simulink model "P702_NI_SoftECU"  (R2019a)
settings: Solver=ode1  StartTime=0.0  StopTime=Inf  FixedStep=0.001  RelTol=1e-3  EnableMultiTasking=on
PreLoadFcn:
  | run '.\VeriStand_BlockSet\NIVeriStandAddPaths.m'
undefined symbols (not defined in the file or in its folder): magnitude
libraries: simulink x83, simulink_extras x1
(part 73 of 76)

== system P702_NI_SoftECU/Output/Subsystem1/CAN_Signal/GWM/RCM/RCMStatusMessage2_FD1_4C ==
  in_port : Inport
  EDRTriggerEvntSync : Terminator
  FirstRowBuckleDriver : Terminator
  FirstRowBuckleMid : Terminator
  FirstRowBucklePsngr : Terminator
  PassRstrnInd_Req : Terminator
  PsngrFmidDetct_D_Actl : Terminator
  PsngrFrntDetct_D_Actl : Terminator
  RILReq : Terminator
  RstrnImpactEvntStatus : Terminator
  RstrnPsngrOn_D_Stat : Terminator
  SecondRowBuckleDriver : Terminator
  SecondRowBuckleMid : Terminator
  SecondRowBucklePsngr : Terminator
  ThirdRowBuckleDriver : Terminator
  ThirdRowBuckleMid : Terminator
  ThirdRowBucklePsngr : Terminator
  bus_selector : BusSelector  OutputSignals=EDRTriggerEvntSync,FirstRowBuckleDriver,FirstRowBuckleMid,FirstRowBucklePsngr,PassRstrnInd_Req,PsngrFmidDetct_D_Actl,PsngrFrntDetct_D_Actl,RILReq,RstrnImpactEvntStatus,RstrnPsngrOn_D_Stat,SecondRowBuckleDriver,SecondRowBuckleMid,SecondRowBucklePsngr,ThirdRowBuckleDriver,ThirdRowBuckleMid,ThirdRowBucklePsngr
  wires:
  in_port/1 -> bus_selector/1  "Subsystem1"
  bus_selector/1 -> EDRTriggerEvntSync/1  "<EDRTriggerEvntSync>"
  bus_selector/2 -> FirstRowBuckleDriver/1  "<FirstRowBuckleDriver>"
  bus_selector/3 -> FirstRowBuckleMid/1  "<FirstRowBuckleMid>"
  bus_selector/4 -> FirstRowBucklePsngr/1  "<FirstRowBucklePsngr>"
  bus_selector/5 -> PassRstrnInd_Req/1  "<PassRstrnInd_Req>"
  bus_selector/6 -> PsngrFmidDetct_D_Actl/1  "<PsngrFmidDetct_D_Actl>"
  bus_selector/7 -> PsngrFrntDetct_D_Actl/1  "<PsngrFrntDetct_D_Actl>"
  bus_selector/8 -> RILReq/1  "<RILReq>"
  bus_selector/9 -> RstrnImpactEvntStatus/1  "<RstrnImpactEvntStatus>"
  bus_selector/10 -> RstrnPsngrOn_D_Stat/1  "<RstrnPsngrOn_D_Stat>"
  bus_selector/11 -> SecondRowBuckleDriver/1  "<SecondRowBuckleDriver>"
  bus_selector/12 -> SecondRowBuckleMid/1  "<SecondRowBuckleMid>"
  bus_selector/13 -> SecondRowBucklePsngr/1  "<SecondRowBucklePsngr>"
  bus_selector/14 -> ThirdRowBuckleDriver/1  "<ThirdRowBuckleDriver>"
  bus_selector/15 -> ThirdRowBuckleMid/1  "<ThirdRowBuckleMid>"
  bus_selector/16 -> ThirdRowBucklePsngr/1  "<ThirdRowBucklePsngr>"

== system P702_NI_SoftECU/Output/Subsystem1/CAN_Signal/GWM/SCCM/Steering_Data_FD1_83 ==
  in_port : Inport
  AccButtnGapDecPress : Terminator
  AccButtnGapIncPress : Terminator
  AccButtnGapTogglePress : Terminator
  AhbStat_B_Dsply : Terminator
  AslButtnOnOffCnclPress : Terminator
  AslButtnOnOffPress : Terminator
  CcAslButtnCnclPress : Terminator
  CcAslButtnCnclResPress : Terminator
  CcAslButtnDeny_B_Actl : Terminator
  CcAslButtnIndxDecPress : Terminator
  CcAslButtnIndxIncPress : Terminator
  CcAslButtnOffCnclPress : Terminator
  CcAslButtnOnOffCncl : Terminator
  CcAslButtnOnPress : Terminator
  CcAslButtnResDecPress : Terminator
  CcAslButtnResIncPress : Terminator
  CcAslButtnSetDecPress : Terminator
  CcAslButtnSetIncPress : Terminator
  CcAslButtnSetPress : Terminator
  CcAsllButtnResPress : Terminator
  CcButtnOffPress : Terminator
  CcButtnOnOffCnclPress : Terminator
  CcButtnOnOffPress : Terminator
  CcButtnOnPress : Terminator
  HeadLghtHiCtrl_D_RqAhb : Terminator
  HeadLghtHiFlash_D_Actl : Terminator
  HeadLghtHiFlash_D_Stat : Terminator
  HeadLghtHiOn_B_StatAhb : Terminator
  LaSwtchPos_D_Stat : Terminator
  LghtAmb_D_Sns : Terminator
  TjaButtnOnOffPress : Terminator
  TurnLghtSwtch_D_Stat : Terminator
  WiprFrontSwtch_D_Stat : Terminator
  WiprFront_D_Stat : Terminator
  bus_selector : BusSelector  OutputSignals=AccButtnGapDecPress,AccButtnGapIncPress,AccButtnGapTogglePress,AhbStat_B_Dsply,AslButtnOnOffCnclPress,AslButtnOnOffPress,CcAslButtnCnclPress,CcAslButtnCnclResPress,CcAslButtnDeny_B_Actl,CcAslButtnIndxDecPress,CcAslButtnIndxIncPress,CcAslButtnOffCnclPress,CcAslButtnOnOffCncl,CcAslButtnOnPress,CcAslButtnResDecPress,CcAslButtnResIncPress,CcAslButtnSetDecPress,CcAslButtnSetIncPress,CcAslButtnSetPress,CcAsllButtnResPress,CcButtnOffPress,CcButtnOnOffCnclPress,CcButtnOnOffPress,CcButtnOnPress,HeadLghtHiCtrl_D_RqAhb,HeadLghtHiFlash_D_Actl,HeadLghtHiFlash_D_Stat,HeadLghtHiOn_B_StatAhb,LaSwtchPos_D_Stat,LghtAmb_D_Sns,TjaButtnOnOffPress,TurnLghtSwtch_D_Stat,WiprFrontSwtch_D_Stat,WiprFront_D_Stat
  wires:
  in_port/1 -> bus_selector/1  "Subsystem1"
  bus_selector/1 -> AccButtnGapDecPress/1  "<AccButtnGapDecPress>"
  bus_selector/2 -> AccButtnGapIncPress/1  "<AccButtnGapIncPress>"
  bus_selector/3 -> AccButtnGapTogglePress/1  "<AccButtnGapTogglePress>"
  bus_selector/4 -> AhbStat_B_Dsply/1  "<AhbStat_B_Dsply>"
  bus_selector/5 -> AslButtnOnOffCnclPress/1  "<AslButtnOnOffCnclPress>"
  bus_selector/6 -> AslButtnOnOffPress/1  "<AslButtnOnOffPress>"
  bus_selector/7 -> CcAslButtnCnclPress/1  "<CcAslButtnCnclPress>"
  bus_selector/8 -> CcAslButtnCnclResPress/1  "<CcAslButtnCnclResPress>"
  bus_selector/9 -> CcAslButtnDeny_B_Actl/1  "<CcAslButtnDeny_B_Actl>"
  bus_selector/10 -> CcAslButtnIndxDecPress/1  "<CcAslButtnIndxDecPress>"
  bus_selector/11 -> CcAslButtnIndxIncPress/1  "<CcAslButtnIndxIncPress>"
  bus_selector/12 -> CcAslButtnOffCnclPress/1  "<CcAslButtnOffCnclPress>"
  bus_selector/13 -> CcAslButtnOnOffCncl/1  "<CcAslButtnOnOffCncl>"
  bus_selector/14 -> CcAslButtnOnPress/1  "<CcAslButtnOnPress>"
  bus_selector/15 -> CcAslButtnResDecPress/1  "<CcAslButtnResDecPress>"
  bus_selector/16 -> CcAslButtnResIncPress/1  "<CcAslButtnResIncPress>"
  bus_selector/17 -> CcAslButtnSetDecPress/1  "<CcAslButtnSetDecPress>"
  bus_selector/18 -> CcAslButtnSetIncPress/1  "<CcAslButtnSetIncPress>"
  bus_selector/19 -> CcAslButtnSetPress/1  "<CcAslButtnSetPress>"
  bus_selector/20 -> CcAsllButtnResPress/1  "<CcAsllButtnResPress>"
  bus_selector/21 -> CcButtnOffPress/1  "<CcButtnOffPress>"
  bus_selector/22 -> CcButtnOnOffCnclPress/1  "<CcButtnOnOffCnclPress>"
  bus_selector/23 -> CcButtnOnOffPress/1  "<CcButtnOnOffPress>"
  bus_selector/24 -> CcButtnOnPress/1  "<CcButtnOnPress>"
  bus_selector/25 -> HeadLghtHiCtrl_D_RqAhb/1  "<HeadLghtHiCtrl_D_RqAhb>"
  bus_selector/26 -> HeadLghtHiFlash_D_Actl/1  "<HeadLghtHiFlash_D_Actl>"
  bus_selector/27 -> HeadLghtHiFlash_D_Stat/1  "<HeadLghtHiFlash_D_Stat>"
  bus_selector/28 -> HeadLghtHiOn_B_StatAhb/1  "<HeadLghtHiOn_B_StatAhb>"
  bus_selector/29 -> LaSwtchPos_D_Stat/1  "<LaSwtchPos_D_Stat>"
  bus_selector/30 -> LghtAmb_D_Sns/1  "<LghtAmb_D_Sns>"
  bus_selector/31 -> TjaButtnOnOffPress/1  "<TjaButtnOnOffPress>"
  bus_selector/32 -> TurnLghtSwtch_D_Stat/1  "<TurnLghtSwtch_D_Stat>"
  bus_selector/33 -> WiprFrontSwtch_D_Stat/1  "<WiprFrontSwtch_D_Stat>"
  bus_selector/34 -> WiprFront_D_Stat/1  "<WiprFront_D_Stat>"

== system P702_NI_SoftECU/Output/Subsystem1/CAN_Signal/GWM/SCCM/Steering_Wheel_Data2_FD1_81 ==
  in_port : Inport
  SelDrvMdeDec_B_RqDrv : Terminator
  SelDrvMdeInc_B_RqDrv : Terminator
  SelDrvMdeSwtch_D_Stat4 : Terminator
  SteEffortInc_B_RqDrv : Terminator
  SteWhlSwtchBack_B_Stat : Terminator
  SteWhlSwtchDown_B_Stat : Terminator
  SteWhlSwtchHome_B_Stat : Terminator
  SteWhlSwtchHud_B_Stat : Terminator
  SteWhlSwtchInfo_B_Stat : Terminator
  SteWhlSwtchIod_B_Stat : Terminator
  SteWhlSwtchLeft_B_Stat : Terminator
  SteWhlSwtchMed_B_Stat : Terminator
  SteWhlSwtchMenu_B_Stat : Terminator
  SteWhlSwtchNav_B_Stat : Terminator
  SteWhlSwtchOk_B_Stat : Terminator
  SteWhlSwtchPhon_B_Stat : Terminator
  SteWhlSwtchRght_B_Stat : Terminator
  SteWhlSwtchSet_B_Stat : Terminator
  SteWhlSwtchUp_B_Stat : Terminator
  SteWhlSwtchView_B_Stat : Terminator
  SuspDampInc_B_RqDrv : Terminator
  bus_selector : BusSelector  OutputSignals=SelDrvMdeDec_B_RqDrv,SelDrvMdeInc_B_RqDrv,SelDrvMdeSwtch_D_Stat4,SteEffortInc_B_RqDrv,SteWhlSwtchBack_B_Stat,SteWhlSwtchDown_B_Stat,SteWhlSwtchHome_B_Stat,SteWhlSwtchHud_B_Stat,SteWhlSwtchInfo_B_Stat,SteWhlSwtchIod_B_Stat,SteWhlSwtchLeft_B_Stat,SteWhlSwtchMed_B_Stat,SteWhlSwtchMenu_B_Stat,SteWhlSwtchNav_B_Stat,SteWhlSwtchOk_B_Stat,SteWhlSwtchPhon_B_Stat,SteWhlSwtchRght_B_Stat,SteWhlSwtchSet_B_Stat,SteWhlSwtchUp_B_Stat,SteWhlSwtchView_B_Stat,SuspDampInc_B_RqDrv
  wires:
  in_port/1 -> bus_selector/1  "Subsystem1"
  bus_selector/1 -> SelDrvMdeDec_B_RqDrv/1  "<SelDrvMdeDec_B_RqDrv>"
  bus_selector/2 -> SelDrvMdeInc_B_RqDrv/1  "<SelDrvMdeInc_B_RqDrv>"
  bus_selector/3 -> SelDrvMdeSwtch_D_Stat4/1  "<SelDrvMdeSwtch_D_Stat4>"
  bus_selector/4 -> SteEffortInc_B_RqDrv/1  "<SteEffortInc_B_RqDrv>"
  bus_selector/5 -> SteWhlSwtchBack_B_Stat/1  "<SteWhlSwtchBack_B_Stat>"
  bus_selector/6 -> SteWhlSwtchDown_B_Stat/1  "<SteWhlSwtchDown_B_Stat>"
  bus_selector/7 -> SteWhlSwtchHome_B_Stat/1  "<SteWhlSwtchHome_B_Stat>"
  bus_selector/8 -> SteWhlSwtchHud_B_Stat/1  "<SteWhlSwtchHud_B_Stat>"
  bus_selector/9 -> SteWhlSwtchInfo_B_Stat/1  "<SteWhlSwtchInfo_B_Stat>"
  bus_selector/10 -> SteWhlSwtchIod_B_Stat/1  "<SteWhlSwtchIod_B_Stat>"
  bus_selector/11 -> SteWhlSwtchLeft_B_Stat/1  "<SteWhlSwtchLeft_B_Stat>"
  bus_selector/12 -> SteWhlSwtchMed_B_Stat/1  "<SteWhlSwtchMed_B_Stat>"
  bus_selector/13 -> SteWhlSwtchMenu_B_Stat/1  "<SteWhlSwtchMenu_B_Stat>"
  bus_selector/14 -> SteWhlSwtchNav_B_Stat/1  "<SteWhlSwtchNav_B_Stat>"
  bus_selector/15 -> SteWhlSwtchOk_B_Stat/1  "<SteWhlSwtchOk_B_Stat>"
  bus_selector/16 -> SteWhlSwtchPhon_B_Stat/1  "<SteWhlSwtchPhon_B_Stat>"
  bus_selector/17 -> SteWhlSwtchRght_B_Stat/1  "<SteWhlSwtchRght_B_Stat>"
  bus_selector/18 -> SteWhlSwtchSet_B_Stat/1  "<SteWhlSwtchSet_B_Stat>"
  bus_selector/19 -> SteWhlSwtchUp_B_Stat/1  "<SteWhlSwtchUp_B_Stat>"
  bus_selector/20 -> SteWhlSwtchView_B_Stat/1  "<SteWhlSwtchView_B_Stat>"
  bus_selector/21 -> SuspDampInc_B_RqDrv/1  "<SuspDampInc_B_RqDrv>"

== system P702_NI_SoftECU/Output/Subsystem1/CAN_Signal/GWM/Tester//AutoSar/GWM_AutoSar_NetMgmt_FD1 ==
  in_port : Inport
  GWM_AutoSarNMControl : Terminator
  GWM_AutoSarNMNodeId : Terminator
  GWM_AutoSarNMReserved{1..4} (4 alike) : Terminator
  GWM_GWNMProxy : Terminator
  GWM_GWOnBoardTester : Terminator
  bus_selector : BusSelector  OutputSignals=GWM_AutoSarNMControl,GWM_AutoSarNMNodeId,GWM_AutoSarNMReserved1,GWM_AutoSarNMReserved2,GWM_AutoSarNMReserved3,GWM_AutoSarNMReserved4,GWM_GWNMProxy,GWM_GWOnBoardTester
  wires:
  in_port/1 -> bus_selector/1  "Subsystem1"
  bus_selector/1 -> GWM_AutoSarNMControl/1  "<GWM_AutoSarNMControl>"
  bus_selector/2 -> GWM_AutoSarNMNodeId/1  "<GWM_AutoSarNMNodeId>"
  bus_selector/3 -> GWM_AutoSarNMReserved1/1  "<GWM_AutoSarNMReserved1>"
  bus_selector/4 -> GWM_AutoSarNMReserved2/1  "<GWM_AutoSarNMReserved2>"
  bus_selector/5 -> GWM_AutoSarNMReserved3/1  "<GWM_AutoSarNMReserved3>"
  bus_selector/6 -> GWM_AutoSarNMReserved4/1  "<GWM_AutoSarNMReserved4>"
  bus_selector/7 -> GWM_GWNMProxy/1  "<GWM_GWNMProxy>"
  bus_selector/8 -> GWM_GWOnBoardTester/1  "<GWM_GWOnBoardTester>"

== system P702_NI_SoftECU/Output/Subsystem1/CAN_Signal/GWM/Tester//AutoSar/TesterPhysicalResGWM_FD1 ==
  in_port : Inport
  TesterPhysicalResGWM_F1 : Terminator
  bus_selector : BusSelector  OutputSignals=TesterPhysicalResGWM_F1
  wires:
  in_port/1 -> bus_selector/1  "Subsystem1"
  bus_selector/1 -> TesterPhysicalResGWM_F1/1  "<TesterPhysicalResGWM_F1>"

== system P702_NI_SoftECU/Output/Subsystem1/To_NI_HIL/SRR_L/FL_SOD/SRR_FL_001 ==
  in_port : Inport
  SRR_FL_CAN_DET_AMPLITUDE_01 : Terminator
  SRR_FL_CAN_DET_AZIMUTH_01 : Terminator
  SRR_FL_CAN_DET_ELEVATION_01 : Terminator
  SRR_FL_CAN_DET_RANGE_01 : Terminator
  SRR_FL_CAN_DET_RANGE_RATE_01 : Terminator
  SRR_FL_CAN_DET_SUPER_RES_TARGET_01 : Terminator
  SRR_FL_CAN_DET_VALID_LEVEL_01 : Terminator
  bus_selector : BusSelector  OutputSignals=SRR_FL_CAN_DET_RANGE_01,SRR_FL_CAN_DET_RANGE_RATE_01,SRR_FL_CAN_DET_AZIMUTH_01,SRR_FL_CAN_DET_ELEVATION_01,SRR_FL_CAN_DET_SUPER_RES_TARGET_01,SRR_FL_CAN_DET_AMPLITUDE_01,SRR_FL_CAN_DET_VALID_LEVEL_01
  wires:
  in_port/1 -> bus_selector/1  "Subsystem1"
  bus_selector/1 -> SRR_FL_CAN_DET_RANGE_01/1  "<SRR_FL_CAN_DET_RANGE_01>"
  bus_selector/2 -> SRR_FL_CAN_DET_RANGE_RATE_01/1  "<SRR_FL_CAN_DET_RANGE_RATE_01>"
  bus_selector/3 -> SRR_FL_CAN_DET_AZIMUTH_01/1  "<SRR_FL_CAN_DET_AZIMUTH_01>"
  bus_selector/4 -> SRR_FL_CAN_DET_ELEVATION_01/1  "<SRR_FL_CAN_DET_ELEVATION_01>"
  bus_selector/5 -> SRR_FL_CAN_DET_SUPER_RES_TARGET_01/1  "<SRR_FL_CAN_DET_SUPER_RES_TARGET_01>"
  bus_selector/6 -> SRR_FL_CAN_DET_AMPLITUDE_01/1  "<SRR_FL_CAN_DET_AMPLITUDE_01>"
  bus_selector/7 -> SRR_FL_CAN_DET_VALID_LEVEL_01/1  "<SRR_FL_CAN_DET_VALID_LEVEL_01>"

== system P702_NI_SoftECU/Output/Subsystem1/To_NI_HIL/SRR_L/FL_SOD/SRR_FL_002 ==
  in_port : Inport
  SRR_FL_CAN_DET_AMPLITUDE_02 : Terminator
  SRR_FL_CAN_DET_AZIMUTH_02 : Terminator
  SRR_FL_CAN_DET_ELEVATION_02 : Terminator
  SRR_FL_CAN_DET_RANGE_02 : Terminator
  SRR_FL_CAN_DET_RANGE_RATE_02 : Terminator
  SRR_FL_CAN_DET_SUPER_RES_TARGET_02 : Terminator
  SRR_FL_CAN_DET_VALID_LEVEL_02 : Terminator
  bus_selector : BusSelector  OutputSignals=SRR_FL_CAN_DET_RANGE_02,SRR_FL_CAN_DET_RANGE_RATE_02,SRR_FL_CAN_DET_AZIMUTH_02,SRR_FL_CAN_DET_ELEVATION_02,SRR_FL_CAN_DET_SUPER_RES_TARGET_02,SRR_FL_CAN_DET_AMPLITUDE_02,SRR_FL_CAN_DET_VALID_LEVEL_02
  wires:
  in_port/1 -> bus_selector/1  "Subsystem1"
  bus_selector/1 -> SRR_FL_CAN_DET_RANGE_02/1  "<SRR_FL_CAN_DET_RANGE_02>"
  bus_selector/2 -> SRR_FL_CAN_DET_RANGE_RATE_02/1  "<SRR_FL_CAN_DET_RANGE_RATE_02>"
  bus_selector/3 -> SRR_FL_CAN_DET_AZIMUTH_02/1  "<SRR_FL_CAN_DET_AZIMUTH_02>"
  bus_selector/4 -> SRR_FL_CAN_DET_ELEVATION_02/1  "<SRR_FL_CAN_DET_ELEVATION_02>"
  bus_selector/5 -> SRR_FL_CAN_DET_SUPER_RES_TARGET_02/1  "<SRR_FL_CAN_DET_SUPER_RES_TARGET_02>"
  bus_selector/6 -> SRR_FL_CAN_DET_AMPLITUDE_02/1  "<SRR_FL_CAN_DET_AMPLITUDE_02>"
  bus_selector/7 -> SRR_FL_CAN_DET_VALID_LEVEL_02/1  "<SRR_FL_CAN_DET_VALID_LEVEL_02>"

== system P702_NI_SoftECU/Output/Subsystem1/To_NI_HIL/SRR_L/FL_SOD/SRR_FL_003 ==
  in_port : Inport
  SRR_FL_CAN_DET_AMPLITUDE_03 : Terminator
  SRR_FL_CAN_DET_AZIMUTH_03 : Terminator
  SRR_FL_CAN_DET_ELEVATION_03 : Terminator
  SRR_FL_CAN_DET_RANGE_03 : Terminator
  SRR_FL_CAN_DET_RANGE_RATE_03 : Terminator
  SRR_FL_CAN_DET_SUPER_RES_TARGET_03 : Terminator
  SRR_FL_CAN_DET_VALID_LEVEL_03 : Terminator
  bus_selector : BusSelector  OutputSignals=SRR_FL_CAN_DET_RANGE_03,SRR_FL_CAN_DET_RANGE_RATE_03,SRR_FL_CAN_DET_AZIMUTH_03,SRR_FL_CAN_DET_ELEVATION_03,SRR_FL_CAN_DET_SUPER_RES_TARGET_03,SRR_FL_CAN_DET_AMPLITUDE_03,SRR_FL_CAN_DET_VALID_LEVEL_03
  wires:
  in_port/1 -> bus_selector/1  "Subsystem1"
  bus_selector/1 -> SRR_FL_CAN_DET_RANGE_03/1  "<SRR_FL_CAN_DET_RANGE_03>"
  bus_selector/2 -> SRR_FL_CAN_DET_RANGE_RATE_03/1  "<SRR_FL_CAN_DET_RANGE_RATE_03>"
  bus_selector/3 -> SRR_FL_CAN_DET_AZIMUTH_03/1  "<SRR_FL_CAN_DET_AZIMUTH_03>"
  bus_selector/4 -> SRR_FL_CAN_DET_ELEVATION_03/1  "<SRR_FL_CAN_DET_ELEVATION_03>"
  bus_selector/5 -> SRR_FL_CAN_DET_SUPER_RES_TARGET_03/1  "<SRR_FL_CAN_DET_SUPER_RES_TARGET_03>"
  bus_selector/6 -> SRR_FL_CAN_DET_AMPLITUDE_03/1  "<SRR_FL_CAN_DET_AMPLITUDE_03>"
  bus_selector/7 -> SRR_FL_CAN_DET_VALID_LEVEL_03/1  "<SRR_FL_CAN_DET_VALID_LEVEL_03>"

== system P702_NI_SoftECU/Output/Subsystem1/To_NI_HIL/SRR_L/RL_SOD/SRR_RL_001 ==
  in_port : Inport
  SRR_RL_CAN_DET_AMPLITUDE_01 : Terminator
  SRR_RL_CAN_DET_AZIMUTH_01 : Terminator
  SRR_RL_CAN_DET_ELEVATION_01 : Terminator
  SRR_RL_CAN_DET_RANGE_01 : Terminator
  SRR_RL_CAN_DET_RANGE_RATE_01 : Terminator
  SRR_RL_CAN_DET_SUPER_RES_TARGET_01 : Terminator
  SRR_RL_CAN_DET_VALID_LEVEL_01 : Terminator
  bus_selector : BusSelector  OutputSignals=SRR_RL_CAN_DET_RANGE_01,SRR_RL_CAN_DET_RANGE_RATE_01,SRR_RL_CAN_DET_AZIMUTH_01,SRR_RL_CAN_DET_ELEVATION_01,SRR_RL_CAN_DET_SUPER_RES_TARGET_01,SRR_RL_CAN_DET_AMPLITUDE_01,SRR_RL_CAN_DET_VALID_LEVEL_01
  wires:
  in_port/1 -> bus_selector/1  "Subsystem1"
  bus_selector/1 -> SRR_RL_CAN_DET_RANGE_01/1  "<SRR_RL_CAN_DET_RANGE_01>"
  bus_selector/2 -> SRR_RL_CAN_DET_RANGE_RATE_01/1  "<SRR_RL_CAN_DET_RANGE_RATE_01>"
  bus_selector/3 -> SRR_RL_CAN_DET_AZIMUTH_01/1  "<SRR_RL_CAN_DET_AZIMUTH_01>"
  bus_selector/4 -> SRR_RL_CAN_DET_ELEVATION_01/1  "<SRR_RL_CAN_DET_ELEVATION_01>"
  bus_selector/5 -> SRR_RL_CAN_DET_SUPER_RES_TARGET_01/1  "<SRR_RL_CAN_DET_SUPER_RES_TARGET_01>"
  bus_selector/6 -> SRR_RL_CAN_DET_AMPLITUDE_01/1  "<SRR_RL_CAN_DET_AMPLITUDE_01>"
  bus_selector/7 -> SRR_RL_CAN_DET_VALID_LEVEL_01/1  "<SRR_RL_CAN_DET_VALID_LEVEL_01>"

== system P702_NI_SoftECU/Output/Subsystem1/To_NI_HIL/SRR_L/RL_SOD/SRR_RL_002 ==
  in_port : Inport
  SRR_RL_CAN_DET_AMPLITUDE_02 : Terminator
  SRR_RL_CAN_DET_AZIMUTH_02 : Terminator
  SRR_RL_CAN_DET_ELEVATION_02 : Terminator
  SRR_RL_CAN_DET_RANGE_02 : Terminator
  SRR_RL_CAN_DET_RANGE_RATE_02 : Terminator
  SRR_RL_CAN_DET_SUPER_RES_TARGET_02 : Terminator
  SRR_RL_CAN_DET_VALID_LEVEL_02 : Terminator
  bus_selector : BusSelector  OutputSignals=SRR_RL_CAN_DET_RANGE_02,SRR_RL_CAN_DET_RANGE_RATE_02,SRR_RL_CAN_DET_AZIMUTH_02,SRR_RL_CAN_DET_ELEVATION_02,SRR_RL_CAN_DET_SUPER_RES_TARGET_02,SRR_RL_CAN_DET_AMPLITUDE_02,SRR_RL_CAN_DET_VALID_LEVEL_02
  wires:
  in_port/1 -> bus_selector/1  "Subsystem1"
  bus_selector/1 -> SRR_RL_CAN_DET_RANGE_02/1  "<SRR_RL_CAN_DET_RANGE_02>"
  bus_selector/2 -> SRR_RL_CAN_DET_RANGE_RATE_02/1  "<SRR_RL_CAN_DET_RANGE_RATE_02>"
  bus_selector/3 -> SRR_RL_CAN_DET_AZIMUTH_02/1  "<SRR_RL_CAN_DET_AZIMUTH_02>"
  bus_selector/4 -> SRR_RL_CAN_DET_ELEVATION_02/1  "<SRR_RL_CAN_DET_ELEVATION_02>"
  bus_selector/5 -> SRR_RL_CAN_DET_SUPER_RES_TARGET_02/1  "<SRR_RL_CAN_DET_SUPER_RES_TARGET_02>"
  bus_selector/6 -> SRR_RL_CAN_DET_AMPLITUDE_02/1  "<SRR_RL_CAN_DET_AMPLITUDE_02>"
  bus_selector/7 -> SRR_RL_CAN_DET_VALID_LEVEL_02/1  "<SRR_RL_CAN_DET_VALID_LEVEL_02>"

== system P702_NI_SoftECU/Output/Subsystem1/To_NI_HIL/SRR_L/RL_SOD/SRR_RL_003 ==
  in_port : Inport
  SRR_RL_CAN_DET_AMPLITUDE_03 : Terminator
  SRR_RL_CAN_DET_AZIMUTH_03 : Terminator
  SRR_RL_CAN_DET_ELEVATION_03 : Terminator
  SRR_RL_CAN_DET_RANGE_03 : Terminator
  SRR_RL_CAN_DET_RANGE_RATE_03 : Terminator
  SRR_RL_CAN_DET_SUPER_RES_TARGET_03 : Terminator
  SRR_RL_CAN_DET_VALID_LEVEL_03 : Terminator
  bus_selector : BusSelector  OutputSignals=SRR_RL_CAN_DET_RANGE_03,SRR_RL_CAN_DET_RANGE_RATE_03,SRR_RL_CAN_DET_AZIMUTH_03,SRR_RL_CAN_DET_ELEVATION_03,SRR_RL_CAN_DET_SUPER_RES_TARGET_03,SRR_RL_CAN_DET_AMPLITUDE_03,SRR_RL_CAN_DET_VALID_LEVEL_03
  wires:
  in_port/1 -> bus_selector/1  "Subsystem1"
  bus_selector/1 -> SRR_RL_CAN_DET_RANGE_03/1  "<SRR_RL_CAN_DET_RANGE_03>"
  bus_selector/2 -> SRR_RL_CAN_DET_RANGE_RATE_03/1  "<SRR_RL_CAN_DET_RANGE_RATE_03>"
  bus_selector/3 -> SRR_RL_CAN_DET_AZIMUTH_03/1  "<SRR_RL_CAN_DET_AZIMUTH_03>"
  bus_selector/4 -> SRR_RL_CAN_DET_ELEVATION_03/1  "<SRR_RL_CAN_DET_ELEVATION_03>"
  bus_selector/5 -> SRR_RL_CAN_DET_SUPER_RES_TARGET_03/1  "<SRR_RL_CAN_DET_SUPER_RES_TARGET_03>"
  bus_selector/6 -> SRR_RL_CAN_DET_AMPLITUDE_03/1  "<SRR_RL_CAN_DET_AMPLITUDE_03>"
  bus_selector/7 -> SRR_RL_CAN_DET_VALID_LEVEL_03/1  "<SRR_RL_CAN_DET_VALID_LEVEL_03>"

== system P702_NI_SoftECU/Output/Subsystem1/To_NI_HIL/SRR_R/FR_SOD/SRR_FR_001 ==
  in_port : Inport
  SRR_FR_CAN_DET_AMPLITUDE_01 : Terminator
  SRR_FR_CAN_DET_AZIMUTH_01 : Terminator
  SRR_FR_CAN_DET_ELEVATION_01 : Terminator
  SRR_FR_CAN_DET_RANGE_01 : Terminator
  SRR_FR_CAN_DET_RANGE_RATE_01 : Terminator
  SRR_FR_CAN_DET_SUPER_RES_TARGET_01 : Terminator
  SRR_FR_CAN_DET_VALID_LEVEL_01 : Terminator
  bus_selector : BusSelector  OutputSignals=SRR_FR_CAN_DET_RANGE_01,SRR_FR_CAN_DET_RANGE_RATE_01,SRR_FR_CAN_DET_AZIMUTH_01,SRR_FR_CAN_DET_ELEVATION_01,SRR_FR_CAN_DET_SUPER_RES_TARGET_01,SRR_FR_CAN_DET_AMPLITUDE_01,SRR_FR_CAN_DET_VALID_LEVEL_01
  wires:
  in_port/1 -> bus_selector/1  "Subsystem1"
  bus_selector/1 -> SRR_FR_CAN_DET_RANGE_01/1  "<SRR_FR_CAN_DET_RANGE_01>"
  bus_selector/2 -> SRR_FR_CAN_DET_RANGE_RATE_01/1  "<SRR_FR_CAN_DET_RANGE_RATE_01>"
  bus_selector/3 -> SRR_FR_CAN_DET_AZIMUTH_01/1  "<SRR_FR_CAN_DET_AZIMUTH_01>"
  bus_selector/4 -> SRR_FR_CAN_DET_ELEVATION_01/1  "<SRR_FR_CAN_DET_ELEVATION_01>"
  bus_selector/5 -> SRR_FR_CAN_DET_SUPER_RES_TARGET_01/1  "<SRR_FR_CAN_DET_SUPER_RES_TARGET_01>"
  bus_selector/6 -> SRR_FR_CAN_DET_AMPLITUDE_01/1  "<SRR_FR_CAN_DET_AMPLITUDE_01>"
  bus_selector/7 -> SRR_FR_CAN_DET_VALID_LEVEL_01/1  "<SRR_FR_CAN_DET_VALID_LEVEL_01>"

== system P702_NI_SoftECU/Output/Subsystem1/To_NI_HIL/SRR_R/FR_SOD/SRR_FR_002 ==
  in_port : Inport
  SRR_FR_CAN_DET_AMPLITUDE_02 : Terminator
  SRR_FR_CAN_DET_AZIMUTH_02 : Terminator
  SRR_FR_CAN_DET_ELEVATION_02 : Terminator
  SRR_FR_CAN_DET_RANGE_02 : Terminator
  SRR_FR_CAN_DET_RANGE_RATE_02 : Terminator
  SRR_FR_CAN_DET_SUPER_RES_TARGET_02 : Terminator
  SRR_FR_CAN_DET_VALID_LEVEL_02 : Terminator
  bus_selector : BusSelector  OutputSignals=SRR_FR_CAN_DET_RANGE_02,SRR_FR_CAN_DET_RANGE_RATE_02,SRR_FR_CAN_DET_AZIMUTH_02,SRR_FR_CAN_DET_ELEVATION_02,SRR_FR_CAN_DET_SUPER_RES_TARGET_02,SRR_FR_CAN_DET_AMPLITUDE_02,SRR_FR_CAN_DET_VALID_LEVEL_02
  wires:
  in_port/1 -> bus_selector/1  "Subsystem1"
  bus_selector/1 -> SRR_FR_CAN_DET_RANGE_02/1  "<SRR_FR_CAN_DET_RANGE_02>"
  bus_selector/2 -> SRR_FR_CAN_DET_RANGE_RATE_02/1  "<SRR_FR_CAN_DET_RANGE_RATE_02>"
  bus_selector/3 -> SRR_FR_CAN_DET_AZIMUTH_02/1  "<SRR_FR_CAN_DET_AZIMUTH_02>"
  bus_selector/4 -> SRR_FR_CAN_DET_ELEVATION_02/1  "<SRR_FR_CAN_DET_ELEVATION_02>"
  bus_selector/5 -> SRR_FR_CAN_DET_SUPER_RES_TARGET_02/1  "<SRR_FR_CAN_DET_SUPER_RES_TARGET_02>"
  bus_selector/6 -> SRR_FR_CAN_DET_AMPLITUDE_02/1  "<SRR_FR_CAN_DET_AMPLITUDE_02>"
  bus_selector/7 -> SRR_FR_CAN_DET_VALID_LEVEL_02/1  "<SRR_FR_CAN_DET_VALID_LEVEL_02>"

== system P702_NI_SoftECU/Output/Subsystem1/To_NI_HIL/SRR_R/FR_SOD/SRR_FR_003 ==
  in_port : Inport
  SRR_FR_CAN_DET_AMPLITUDE_03 : Terminator
  SRR_FR_CAN_DET_AZIMUTH_03 : Terminator
  SRR_FR_CAN_DET_ELEVATION_03 : Terminator
  SRR_FR_CAN_DET_RANGE_03 : Terminator
  SRR_FR_CAN_DET_RANGE_RATE_03 : Terminator
  SRR_FR_CAN_DET_SUPER_RES_TARGET_03 : Terminator
  SRR_FR_CAN_DET_VALID_LEVEL_03 : Terminator
  bus_selector : BusSelector  OutputSignals=SRR_FR_CAN_DET_RANGE_03,SRR_FR_CAN_DET_RANGE_RATE_03,SRR_FR_CAN_DET_AZIMUTH_03,SRR_FR_CAN_DET_ELEVATION_03,SRR_FR_CAN_DET_SUPER_RES_TARGET_03,SRR_FR_CAN_DET_AMPLITUDE_03,SRR_FR_CAN_DET_VALID_LEVEL_03
  wires:
  in_port/1 -> bus_selector/1  "Subsystem1"
  bus_selector/1 -> SRR_FR_CAN_DET_RANGE_03/1  "<SRR_FR_CAN_DET_RANGE_03>"
  bus_selector/2 -> SRR_FR_CAN_DET_RANGE_RATE_03/1  "<SRR_FR_CAN_DET_RANGE_RATE_03>"
  bus_selector/3 -> SRR_FR_CAN_DET_AZIMUTH_03/1  "<SRR_FR_CAN_DET_AZIMUTH_03>"
  bus_selector/4 -> SRR_FR_CAN_DET_ELEVATION_03/1  "<SRR_FR_CAN_DET_ELEVATION_03>"
  bus_selector/5 -> SRR_FR_CAN_DET_SUPER_RES_TARGET_03/1  "<SRR_FR_CAN_DET_SUPER_RES_TARGET_03>"
  bus_selector/6 -> SRR_FR_CAN_DET_AMPLITUDE_03/1  "<SRR_FR_CAN_DET_AMPLITUDE_03>"
  bus_selector/7 -> SRR_FR_CAN_DET_VALID_LEVEL_03/1  "<SRR_FR_CAN_DET_VALID_LEVEL_03>"

== system P702_NI_SoftECU/Output/Subsystem1/To_NI_HIL/SRR_R/RR_SOD/SRR_RR_001 ==
  in_port : Inport
  SRR_RR_CAN_DET_AMPLITUDE_01 : Terminator
  SRR_RR_CAN_DET_AZIMUTH_01 : Terminator
  SRR_RR_CAN_DET_ELEVATION_01 : Terminator
  SRR_RR_CAN_DET_RANGE_01 : Terminator
  SRR_RR_CAN_DET_RANGE_RATE_01 : Terminator
  SRR_RR_CAN_DET_SUPER_RES_TARGET_01 : Terminator
  SRR_RR_CAN_DET_VALID_LEVEL_01 : Terminator
  bus_selector : BusSelector  OutputSignals=SRR_RR_CAN_DET_RANGE_01,SRR_RR_CAN_DET_RANGE_RATE_01,SRR_RR_CAN_DET_AZIMUTH_01,SRR_RR_CAN_DET_ELEVATION_01,SRR_RR_CAN_DET_SUPER_RES_TARGET_01,SRR_RR_CAN_DET_AMPLITUDE_01,SRR_RR_CAN_DET_VALID_LEVEL_01
  wires:
  in_port/1 -> bus_selector/1  "Subsystem1"
  bus_selector/1 -> SRR_RR_CAN_DET_RANGE_01/1  "<SRR_RR_CAN_DET_RANGE_01>"
  bus_selector/2 -> SRR_RR_CAN_DET_RANGE_RATE_01/1  "<SRR_RR_CAN_DET_RANGE_RATE_01>"
  bus_selector/3 -> SRR_RR_CAN_DET_AZIMUTH_01/1  "<SRR_RR_CAN_DET_AZIMUTH_01>"
  bus_selector/4 -> SRR_RR_CAN_DET_ELEVATION_01/1  "<SRR_RR_CAN_DET_ELEVATION_01>"
  bus_selector/5 -> SRR_RR_CAN_DET_SUPER_RES_TARGET_01/1  "<SRR_RR_CAN_DET_SUPER_RES_TARGET_01>"
  bus_selector/6 -> SRR_RR_CAN_DET_AMPLITUDE_01/1  "<SRR_RR_CAN_DET_AMPLITUDE_01>"
  bus_selector/7 -> SRR_RR_CAN_DET_VALID_LEVEL_01/1  "<SRR_RR_CAN_DET_VALID_LEVEL_01>"

== system P702_NI_SoftECU/Output/Subsystem1/To_NI_HIL/SRR_R/RR_SOD/SRR_RR_002 ==
  in_port : Inport
  SRR_RR_CAN_DET_AMPLITUDE_02 : Terminator
  SRR_RR_CAN_DET_AZIMUTH_02 : Terminator
  SRR_RR_CAN_DET_ELEVATION_02 : Terminator
  SRR_RR_CAN_DET_RANGE_02 : Terminator
  SRR_RR_CAN_DET_RANGE_RATE_02 : Terminator
  SRR_RR_CAN_DET_SUPER_RES_TARGET_02 : Terminator
  SRR_RR_CAN_DET_VALID_LEVEL_02 : Terminator
  bus_selector : BusSelector  OutputSignals=SRR_RR_CAN_DET_RANGE_02,SRR_RR_CAN_DET_RANGE_RATE_02,SRR_RR_CAN_DET_AZIMUTH_02,SRR_RR_CAN_DET_ELEVATION_02,SRR_RR_CAN_DET_SUPER_RES_TARGET_02,SRR_RR_CAN_DET_AMPLITUDE_02,SRR_RR_CAN_DET_VALID_LEVEL_02
  wires:
  in_port/1 -> bus_selector/1  "Subsystem1"
  bus_selector/1 -> SRR_RR_CAN_DET_RANGE_02/1  "<SRR_RR_CAN_DET_RANGE_02>"
  bus_selector/2 -> SRR_RR_CAN_DET_RANGE_RATE_02/1  "<SRR_RR_CAN_DET_RANGE_RATE_02>"
  bus_selector/3 -> SRR_RR_CAN_DET_AZIMUTH_02/1  "<SRR_RR_CAN_DET_AZIMUTH_02>"
  bus_selector/4 -> SRR_RR_CAN_DET_ELEVATION_02/1  "<SRR_RR_CAN_DET_ELEVATION_02>"
  bus_selector/5 -> SRR_RR_CAN_DET_SUPER_RES_TARGET_02/1  "<SRR_RR_CAN_DET_SUPER_RES_TARGET_02>"
  bus_selector/6 -> SRR_RR_CAN_DET_AMPLITUDE_02/1  "<SRR_RR_CAN_DET_AMPLITUDE_02>"
  bus_selector/7 -> SRR_RR_CAN_DET_VALID_LEVEL_02/1  "<SRR_RR_CAN_DET_VALID_LEVEL_02>"

== system P702_NI_SoftECU/Output/Subsystem1/To_NI_HIL/SRR_R/RR_SOD/SRR_RR_003 ==
  in_port : Inport
  SRR_RR_CAN_DET_AMPLITUDE_03 : Terminator
  SRR_RR_CAN_DET_AZIMUTH_03 : Terminator
  SRR_RR_CAN_DET_ELEVATION_03 : Terminator
  SRR_RR_CAN_DET_RANGE_03 : Terminator
  SRR_RR_CAN_DET_RANGE_RATE_03 : Terminator
  SRR_RR_CAN_DET_SUPER_RES_TARGET_03 : Terminator
  SRR_RR_CAN_DET_VALID_LEVEL_03 : Terminator
  bus_selector : BusSelector  OutputSignals=SRR_RR_CAN_DET_RANGE_03,SRR_RR_CAN_DET_RANGE_RATE_03,SRR_RR_CAN_DET_AZIMUTH_03,SRR_RR_CAN_DET_ELEVATION_03,SRR_RR_CAN_DET_SUPER_RES_TARGET_03,SRR_RR_CAN_DET_AMPLITUDE_03,SRR_RR_CAN_DET_VALID_LEVEL_03
  wires:
  in_port/1 -> bus_selector/1  "Subsystem1"
  bus_selector/1 -> SRR_RR_CAN_DET_RANGE_03/1  "<SRR_RR_CAN_DET_RANGE_03>"
  bus_selector/2 -> SRR_RR_CAN_DET_RANGE_RATE_03/1  "<SRR_RR_CAN_DET_RANGE_RATE_03>"
  bus_selector/3 -> SRR_RR_CAN_DET_AZIMUTH_03/1  "<SRR_RR_CAN_DET_AZIMUTH_03>"
  bus_selector/4 -> SRR_RR_CAN_DET_ELEVATION_03/1  "<SRR_RR_CAN_DET_ELEVATION_03>"
  bus_selector/5 -> SRR_RR_CAN_DET_SUPER_RES_TARGET_03/1  "<SRR_RR_CAN_DET_SUPER_RES_TARGET_03>"
  bus_selector/6 -> SRR_RR_CAN_DET_AMPLITUDE_03/1  "<SRR_RR_CAN_DET_AMPLITUDE_03>"
  bus_selector/7 -> SRR_RR_CAN_DET_VALID_LEVEL_03/1  "<SRR_RR_CAN_DET_VALID_LEVEL_03>"

== system P702_NI_SoftECU/Output/Subsystem1/To_NI_HIL/Soft_MRR/MRR_Detection/MRR_Detection_001 ==
  in_port : Inport
  CAN_DET_AMPLITUDE_01 : Terminator
  CAN_DET_AZIMUTH_01 : Terminator
  CAN_DET_RANGE_01 : Terminator
  CAN_DET_RANGE_RATE_01 : Terminator
  CAN_DET_VALID_LEVEL_01 : Terminator
  bus_selector : BusSelector  OutputSignals=CAN_DET_RANGE_01,CAN_DET_RANGE_RATE_01,CAN_DET_AZIMUTH_01,CAN_DET_VALID_LEVEL_01,CAN_DET_AMPLITUDE_01
  wires:
  in_port/1 -> bus_selector/1  "Subsystem1"
  bus_selector/1 -> CAN_DET_RANGE_01/1  "<CAN_DET_RANGE_01>"
  bus_selector/2 -> CAN_DET_RANGE_RATE_01/1  "<CAN_DET_RANGE_RATE_01>"
  bus_selector/3 -> CAN_DET_AZIMUTH_01/1  "<CAN_DET_AZIMUTH_01>"
  bus_selector/4 -> CAN_DET_VALID_LEVEL_01/1  "<CAN_DET_VALID_LEVEL_01>"
  bus_selector/5 -> CAN_DET_AMPLITUDE_01/1  "<CAN_DET_AMPLITUDE_01>"

== system P702_NI_SoftECU/Output/Subsystem1/To_NI_HIL/Soft_MRR/MRR_Detection/MRR_Detection_002 ==
  in_port : Inport
  CAN_DET_AMPLITUDE_02 : Terminator
  CAN_DET_AZIMUTH_02 : Terminator
  CAN_DET_RANGE_02 : Terminator
  CAN_DET_RANGE_RATE_02 : Terminator
  CAN_DET_VALID_LEVEL_02 : Terminator
  bus_selector : BusSelector  OutputSignals=CAN_DET_RANGE_02,CAN_DET_RANGE_RATE_02,CAN_DET_AZIMUTH_02,CAN_DET_VALID_LEVEL_02,CAN_DET_AMPLITUDE_02
  wires:
  in_port/1 -> bus_selector/1  "Subsystem1"
  bus_selector/1 -> CAN_DET_RANGE_02/1  "<CAN_DET_RANGE_02>"
  bus_selector/2 -> CAN_DET_RANGE_RATE_02/1  "<CAN_DET_RANGE_RATE_02>"
  bus_selector/3 -> CAN_DET_AZIMUTH_02/1  "<CAN_DET_AZIMUTH_02>"
  bus_selector/4 -> CAN_DET_VALID_LEVEL_02/1  "<CAN_DET_VALID_LEVEL_02>"
  bus_selector/5 -> CAN_DET_AMPLITUDE_02/1  "<CAN_DET_AMPLITUDE_02>"

== system P702_NI_SoftECU/Output/Subsystem1/To_NI_HIL/Soft_MRR/MRR_Detection/MRR_Detection_003 ==
  in_port : Inport
  CAN_DET_AMPLITUDE_03 : Terminator
  CAN_DET_AZIMUTH_03 : Terminator
  CAN_DET_RANGE_03 : Terminator
  CAN_DET_RANGE_RATE_03 : Terminator
  CAN_DET_VALID_LEVEL_03 : Terminator
  bus_selector : BusSelector  OutputSignals=CAN_DET_RANGE_03,CAN_DET_RANGE_RATE_03,CAN_DET_AZIMUTH_03,CAN_DET_VALID_LEVEL_03,CAN_DET_AMPLITUDE_03
  wires:
  in_port/1 -> bus_selector/1  "Subsystem1"
  bus_selector/1 -> CAN_DET_RANGE_03/1  "<CAN_DET_RANGE_03>"
  bus_selector/2 -> CAN_DET_RANGE_RATE_03/1  "<CAN_DET_RANGE_RATE_03>"
  bus_selector/3 -> CAN_DET_AZIMUTH_03/1  "<CAN_DET_AZIMUTH_03>"
  bus_selector/4 -> CAN_DET_VALID_LEVEL_03/1  "<CAN_DET_VALID_LEVEL_03>"
  bus_selector/5 -> CAN_DET_AMPLITUDE_03/1  "<CAN_DET_AMPLITUDE_03>"

== system P702_NI_SoftECU/Output/Subsystem2/CAN_Signal/GWM/GSM/Gear_Shift_by_Wire_2_FD1_168 ==
  GearButtnStuck_B_Actl : Constant  Value=0
  GsmSrvcRqd_B_Rq : Constant  Value=0
  TrnGearPwmFalt_B_Actl : Constant  Value=0
  TrnTrcmPwmSig_D_Actl : Constant  Value=0
  bus_creator : BusCreator  Inputs=4
  out_port : Outport
  wires:
  bus_creator/1 -> out_port/1  "Subsystem2"
  GearButtnStuck_B_Actl/1 -> bus_creator/1  "GearButtnStuck_B_Actl"
  GsmSrvcRqd_B_Rq/1 -> bus_creator/2  "GsmSrvcRqd_B_Rq"
  TrnGearPwmFalt_B_Actl/1 -> bus_creator/3  "TrnGearPwmFalt_B_Actl"
  TrnTrcmPwmSig_D_Actl/1 -> bus_creator/4  "TrnTrcmPwmSig_D_Actl"

== system P702_NI_SoftECU/Output/Subsystem2/CAN_Signal/GWM/GSM/Gear_Shift_by_Wire_FD1_5A ==
  BrkSwtchPos_B_ActlGsm : Constant  Value=0
  DrQltyDrv_D_StatGsm : Constant  Value=0
  GsmGearMsgTxt_D_Rq : Constant  Value=0
  PrkBrkActv_D_RqGsmGear : Constant  Value=0
  TrnBtsiOvrrd_B_Stat : Constant  Value=0
  TrnGearButtn_B_ActlD0 : Constant  Value=0
  TrnGearButtn_B_ActlD1 : Constant  Value=0
  TrnGearButtn_B_ActlD2 : Constant  Value=0
  TrnGearButtn_B_ActlM0 : Constant  Value=0
  TrnGearButtn_B_ActlM1 : Constant  Value=0
  TrnGearButtn_B_ActlM2 : Constant  Value=0
  TrnGearButtn_B_ActlN0 : Constant  Value=0
  TrnGearButtn_B_ActlN1 : Constant  Value=0
  TrnGearButtn_B_ActlN2 : Constant  Value=0
  TrnGearButtn_B_ActlP0 : Constant  Value=0
  TrnGearButtn_B_ActlP1 : Constant  Value=0
  TrnGearButtn_B_ActlP2 : Constant  Value=0
  TrnGearButtn_B_ActlR0 : Constant  Value=0
  TrnGearButtn_B_ActlR1 : Constant  Value=0
  TrnGearButtn_B_ActlR2 : Constant  Value=0
  TrnGearButtn_U_Actl : Constant  Value=0
  TrnGearRqCnt_B_Actl : Constant  Value=0
  TrnGear_D_RqDrv : Constant  Value=0
  TrnGear_No_Cnt : Constant  Value=0
  TrnGear_No_Cs : Constant  Value=0
  TrnGsmNtmState_D_Actl : Constant  Value=0
  TrnRng_D_RqGsm : Constant  Value=0
  TrnValidGearRq_D_Stat : Constant  Value=0
  bus_creator : BusCreator  Inputs=28
  out_port : Outport
  wires:
  bus_creator/1 -> out_port/1  "Subsystem2"
  BrkSwtchPos_B_ActlGsm/1 -> bus_creator/1  "BrkSwtchPos_B_ActlGsm"
  DrQltyDrv_D_StatGsm/1 -> bus_creator/2  "DrQltyDrv_D_StatGsm"
  GsmGearMsgTxt_D_Rq/1 -> bus_creator/3  "GsmGearMsgTxt_D_Rq"
  PrkBrkActv_D_RqGsmGear/1 -> bus_creator/4  "PrkBrkActv_D_RqGsmGear"
  TrnBtsiOvrrd_B_Stat/1 -> bus_creator/5  "TrnBtsiOvrrd_B_Stat"
  TrnGearButtn_B_ActlD0/1 -> bus_creator/6  "TrnGearButtn_B_ActlD0"
  TrnGearButtn_B_ActlD1/1 -> bus_creator/7  "TrnGearButtn_B_ActlD1"
  TrnGearButtn_B_ActlD2/1 -> bus_creator/8  "TrnGearButtn_B_ActlD2"
  TrnGearButtn_B_ActlM0/1 -> bus_creator/9  "TrnGearButtn_B_ActlM0"
  TrnGearButtn_B_ActlM1/1 -> bus_creator/10  "TrnGearButtn_B_ActlM1"
  TrnGearButtn_B_ActlM2/1 -> bus_creator/11  "TrnGearButtn_B_ActlM2"
  TrnGearButtn_B_ActlN0/1 -> bus_creator/12  "TrnGearButtn_B_ActlN0"
  TrnGearButtn_B_ActlN1/1 -> bus_creator/13  "TrnGearButtn_B_ActlN1"
  TrnGearButtn_B_ActlN2/1 -> bus_creator/14  "TrnGearButtn_B_ActlN2"
  TrnGearButtn_B_ActlP0/1 -> bus_creator/15  "TrnGearButtn_B_ActlP0"
  TrnGearButtn_B_ActlP1/1 -> bus_creator/16  "TrnGearButtn_B_ActlP1"
  TrnGearButtn_B_ActlP2/1 -> bus_creator/17  "TrnGearButtn_B_ActlP2"
  TrnGearButtn_B_ActlR0/1 -> bus_creator/18  "TrnGearButtn_B_ActlR0"
  TrnGearButtn_B_ActlR1/1 -> bus_creator/19  "TrnGearButtn_B_ActlR1"
  TrnGearButtn_B_ActlR2/1 -> bus_creator/20  "TrnGearButtn_B_ActlR2"
  TrnGearButtn_U_Actl/1 -> bus_creator/21  "TrnGearButtn_U_Actl"
  TrnGearRqCnt_B_Actl/1 -> bus_creator/22  "TrnGearRqCnt_B_Actl"
  TrnGear_D_RqDrv/1 -> bus_creator/23  "TrnGear_D_RqDrv"
  TrnGear_No_Cnt/1 -> bus_creator/24  "TrnGear_No_Cnt"
  TrnGear_No_Cs/1 -> bus_creator/25  "TrnGear_No_Cs"
  TrnGsmNtmState_D_Actl/1 -> bus_creator/26  "TrnGsmNtmState_D_Actl"
  TrnRng_D_RqGsm/1 -> bus_creator/27  "TrnRng_D_RqGsm"
  TrnValidGearRq_D_Stat/1 -> bus_creator/28  "TrnValidGearRq_D_Stat"

== system P702_NI_SoftECU/Output/Subsystem2/CAN_Signal/GWM/Other_GWMTx/AC_Compressor_Data_FD1 ==
  ElCmprBattSysU_D_Falt : Constant  Value=0
  ElCmprBattURng_D_Falt : Constant  Value=0
  ElCmprInnrErr_D_Falt : Constant  Value=0
  ElCmprLostComm_D_Falt : Constant  Value=0
  ElCmprOverLoad_D_Falt : Constant  Value=0
  ElCmprOverTe_D_Falt : Constant  Value=0
  ElCmprOverTe_D_Stat : Constant  Value=0
  ElCmprPerfErr_D_Falt : Constant  Value=0
  ElCmprSysU_D_Falt : Constant  Value=0
  ElCmprUHi_D_Stat : Constant  Value=0
  ElCmprUHi_U_Actl : Constant  Value=0
  ElCmpr_D_Stat : Constant  Value=0
  ElCmpr_N_Actl : Constant  Value=0
  ElCmpr_Pw_Actl : Constant  Value=0
  bus_creator : BusCreator  Inputs=14
  out_port : Outport
  wires:
  bus_creator/1 -> out_port/1  "Subsystem2"
  ElCmprBattSysU_D_Falt/1 -> bus_creator/1  "ElCmprBattSysU_D_Falt"
  ElCmprBattURng_D_Falt/1 -> bus_creator/2  "ElCmprBattURng_D_Falt"
  ElCmprInnrErr_D_Falt/1 -> bus_creator/3  "ElCmprInnrErr_D_Falt"
  ElCmprLostComm_D_Falt/1 -> bus_creator/4  "ElCmprLostComm_D_Falt"
  ElCmprOverLoad_D_Falt/1 -> bus_creator/5  "ElCmprOverLoad_D_Falt"
  ElCmprOverTe_D_Falt/1 -> bus_creator/6  "ElCmprOverTe_D_Falt"
  ElCmprOverTe_D_Stat/1 -> bus_creator/7  "ElCmprOverTe_D_Stat"
  ElCmprPerfErr_D_Falt/1 -> bus_creator/8  "ElCmprPerfErr_D_Falt"
  ElCmprSysU_D_Falt/1 -> bus_creator/9  "ElCmprSysU_D_Falt"
  ElCmprUHi_D_Stat/1 -> bus_creator/10  "ElCmprUHi_D_Stat"
  ElCmprUHi_U_Actl/1 -> bus_creator/11  "ElCmprUHi_U_Actl"
  ElCmpr_D_Stat/1 -> bus_creator/12  "ElCmpr_D_Stat"
  ElCmpr_N_Actl/1 -> bus_creator/13  "ElCmpr_N_Actl"
  ElCmpr_Pw_Actl/1 -> bus_creator/14  "ElCmpr_Pw_Actl"

== system P702_NI_SoftECU/Output/Subsystem2/CAN_Signal/GWM/Other_GWMTx/AC_Compressor_Req_FD1 ==
  ElCmprEnbl_B_Rq : Constant  Value=0
  ElCmpr_N_Rq : Constant  Value=0
  bus_creator : BusCreator  Inputs=2
  out_port : Outport
  wires:
  bus_creator/1 -> out_port/1  "Subsystem2"
  ElCmprEnbl_B_Rq/1 -> bus_creator/1  "ElCmprEnbl_B_Rq"
  ElCmpr_N_Rq/1 -> bus_creator/2  "ElCmpr_N_Rq"

== system P702_NI_SoftECU/Output/Subsystem2/CAN_Signal/GWM/Other_GWMTx/APIMGPS_Data_Nav_1_FD1 ==
  GPS_Latitude_Degrees : Constant  Value=0
  GPS_Latitude_Min_dec : Constant  Value=0
  GPS_Latitude_Minutes : Constant  Value=0
  GPS_Longitude_Degrees : Constant  Value=0
  GPS_Longitude_Min_dec : Constant  Value=0
  GPS_Longitude_Minutes : Constant  Value=0
  GpsHsphLattSth_D_Actl : Constant  Value=0
  GpsHsphLongEast_D_Actl : Constant  Value=0
  bus_creator : BusCreator  Inputs=8
  out_port : Outport
  wires:
  bus_creator/1 -> out_port/1  "Subsystem2"
  GPS_Latitude_Degrees/1 -> bus_creator/1  "GPS_Latitude_Degrees"
  GPS_Latitude_Min_dec/1 -> bus_creator/2  "GPS_Latitude_Min_dec"
  GPS_Latitude_Minutes/1 -> bus_creator/3  "GPS_Latitude_Minutes"
  GPS_Longitude_Degrees/1 -> bus_creator/4  "GPS_Longitude_Degrees"
  GPS_Longitude_Min_dec/1 -> bus_creator/5  "GPS_Longitude_Min_dec"
  GPS_Longitude_Minutes/1 -> bus_creator/6  "GPS_Longitude_Minutes"
  GpsHsphLattSth_D_Actl/1 -> bus_creator/7  "GpsHsphLattSth_D_Actl"
  GpsHsphLongEast_D_Actl/1 -> bus_creator/8  "GpsHsphLongEast_D_Actl"

== system P702_NI_SoftECU/Output/Subsystem2/CAN_Signal/GWM/Other_GWMTx/APIMGPS_Data_Nav_2_FD1 ==
  GPS_Actual_vs_Infer_pos : Constant  Value=0
  GPS_Compass_direction : Constant  Value=0
  GPS_Pdop : Constant  Value=0
  GPS_UTC_hours : Constant  Value=0
  GPS_UTC_minutes : Constant  Value=0
  GPS_UTC_seconds : Constant  Value=0
  GpsUtcDay_No_Actl : Constant  Value=0
  GpsUtcMnth_No_Actl : Constant  Value=0
  GpsUtcYr_No_Actl : Constant  Value=0
  Gps_B_Falt : Constant  Value=0
  bus_creator : BusCreator  Inputs=10
  out_port : Outport
  wires:
  bus_creator/1 -> out_port/1  "Subsystem2"
  GPS_Actual_vs_Infer_pos/1 -> bus_creator/1  "GPS_Actual_vs_Infer_pos"
  GPS_Compass_direction/1 -> bus_creator/2  "GPS_Compass_direction"
  GPS_Pdop/1 -> bus_creator/3  "GPS_Pdop"
  GPS_UTC_hours/1 -> bus_creator/4  "GPS_UTC_hours"
  GPS_UTC_minutes/1 -> bus_creator/5  "GPS_UTC_minutes"
  GPS_UTC_seconds/1 -> bus_creator/6  "GPS_UTC_seconds"
  GpsUtcDay_No_Actl/1 -> bus_creator/7  "GpsUtcDay_No_Actl"
  GpsUtcMnth_No_Actl/1 -> bus_creator/8  "GpsUtcMnth_No_Actl"
  GpsUtcYr_No_Actl/1 -> bus_creator/9  "GpsUtcYr_No_Actl"
  Gps_B_Falt/1 -> bus_creator/10  "Gps_B_Falt"

== system P702_NI_SoftECU/Output/Subsystem2/CAN_Signal/GWM/Other_GWMTx/APIM_Request_Signals_1_FD1 ==
  ChrgOvrdExitScrn_D_Rq : Constant  Value=0
  EmPrflButtnAssoc_D_Rq : Constant  Value=0
  EmPrflKeyAssoc_D_Rq : Constant  Value=0
  EmPrflNo_D_Rq : Constant  Value=0
  Em_D_Stat : Constant  Value=0
  Rba_D_Rq : Constant  Value=0
  bus_creator : BusCreator  Inputs=6
  out_port : Outport
  wires:
  bus_creator/1 -> out_port/1  "Subsystem2"
  ChrgOvrdExitScrn_D_Rq/1 -> bus_creator/1  "ChrgOvrdExitScrn_D_Rq"
  EmPrflButtnAssoc_D_Rq/1 -> bus_creator/2  "EmPrflButtnAssoc_D_Rq"
  EmPrflKeyAssoc_D_Rq/1 -> bus_creator/3  "EmPrflKeyAssoc_D_Rq"
  EmPrflNo_D_Rq/1 -> bus_creator/4  "EmPrflNo_D_Rq"
  Em_D_Stat/1 -> bus_creator/5  "Em_D_Stat"
  Rba_D_Rq/1 -> bus_creator/6  "Rba_D_Rq"

== system P702_NI_SoftECU/Output/Subsystem2/CAN_Signal/GWM/Other_GWMTx/APIM_Request_Signals_FD1 ==
  CbnCmrtPrefListIndx_Rq : Constant  Value=0
  CbnCmrtPrefLstNmItm_Rq : Constant  Value=0
  ChargePortPwr_Rq : Constant  Value=0
  ChrgStatDsply_D_Rq : Constant  Value=0
  FactoryReset_Rq : Constant  Value=0
  LongTermParking_Rq : Constant  Value=0
  ModemReset_D_Rq : Constant  Value=0
  NextUsageTimeToggle_Rq : Constant  Value=0
  OffPeakTimeSetHR_Rq : Constant  Value=0
  OffPeakTimeSetMin_Rq : Constant  Value=0
  StopStrtDrvMde_B_RqBtn3 : Constant  Value=0
  TCU_ESN_D_Rq : Constant  Value=0
  bus_creator : BusCreator  Inputs=12
  out_port : Outport
  wires:
  bus_creator/1 -> out_port/1  "Subsystem2"
  CbnCmrtPrefListIndx_Rq/1 -> bus_creator/1  "CbnCmrtPrefListIndx_Rq"
  CbnCmrtPrefLstNmItm_Rq/1 -> bus_creator/2  "CbnCmrtPrefLstNmItm_Rq"
  ChargePortPwr_Rq/1 -> bus_creator/3  "ChargePortPwr_Rq"
  ChrgStatDsply_D_Rq/1 -> bus_creator/4  "ChrgStatDsply_D_Rq"
  FactoryReset_Rq/1 -> bus_creator/5  "FactoryReset_Rq"
  LongTermParking_Rq/1 -> bus_creator/6  "LongTermParking_Rq"
  ModemReset_D_Rq/1 -> bus_creator/7  "ModemReset_D_Rq"
  NextUsageTimeToggle_Rq/1 -> bus_creator/8  "NextUsageTimeToggle_Rq"
  OffPeakTimeSetHR_Rq/1 -> bus_creator/9  "OffPeakTimeSetHR_Rq"
  OffPeakTimeSetMin_Rq/1 -> bus_creator/10  "OffPeakTimeSetMin_Rq"
  StopStrtDrvMde_B_RqBtn3/1 -> bus_creator/11  "StopStrtDrvMde_B_RqBtn3"
  TCU_ESN_D_Rq/1 -> bus_creator/12  "TCU_ESN_D_Rq"

== system P702_NI_SoftECU/Output/Subsystem2/CAN_Signal/GWM/Other_GWMTx/APIM_Send_Signals1_FD1 ==
  APIM_ActiveTrackNum_St : Constant  Value=0
  APIM_NumberofTracks_St : Constant  Value=0
  AutoHoldSwtch_D_Stat3 : Constant  Value=0
  CenterStackRing_D_Actl : Constant  Value=0
  ChrgCordUnlock_B_Rq : Constant  Value=0
  TrlrAidCancl_B_Rq : Constant  Value=0
  TrlrAidSetup_D_Stat : Constant  Value=0
  TrlrTrgtAcquire_D_Rq : Constant  Value=0
  ValetMode_D_Stat : Constant  Value=0
  bus_creator : BusCreator  Inputs=9
  out_port : Outport
  wires:
  bus_creator/1 -> out_port/1  "Subsystem2"
  APIM_ActiveTrackNum_St/1 -> bus_creator/1  "APIM_ActiveTrackNum_St"
  APIM_NumberofTracks_St/1 -> bus_creator/2  "APIM_NumberofTracks_St"
  AutoHoldSwtch_D_Stat3/1 -> bus_creator/3  "AutoHoldSwtch_D_Stat3"
  CenterStackRing_D_Actl/1 -> bus_creator/4  "CenterStackRing_D_Actl"
  ChrgCordUnlock_B_Rq/1 -> bus_creator/5  "ChrgCordUnlock_B_Rq"
  TrlrAidCancl_B_Rq/1 -> bus_creator/6  "TrlrAidCancl_B_Rq"
  TrlrAidSetup_D_Stat/1 -> bus_creator/7  "TrlrAidSetup_D_Stat"
  TrlrTrgtAcquire_D_Rq/1 -> bus_creator/8  "TrlrTrgtAcquire_D_Rq"
  ValetMode_D_Stat/1 -> bus_creator/9  "ValetMode_D_Stat"

== system P702_NI_SoftECU/Output/Subsystem2/CAN_Signal/GWM/Other_GWMTx/APIM_Send_Signals_2_FD1 ==
  OnbChrgClearAll_B_Rq : Constant  Value=0
  OnbChrgGoTDelete_B_Rq : Constant  Value=0
  OnbChrgGoTElement_D_Rq : Constant  Value=0
  OnbChrgGoTExtHtr_D_Rq : Constant  Value=0
  OnbChrgGoTHr_T_Rq : Constant  Value=0
  OnbChrgGoTMnte_D_Rq : Constant  Value=0
  OnbChrgGoTOn_D_Rq : Constant  Value=0
  OnbChrgGoTPrcond_D_Rq : Constant  Value=0
  OnbChrgGoTTouch_D_Rq : Constant  Value=0
  OnbChrgGoTUpdate_B_Rq : Constant  Value=0
  OtaTrg_D_Stat : Constant  Value=0
  PaakMyKey_D_Rq : Constant  Value=0
  TCU_Final_Actvtn_St : Constant  Value=0
  TCU_Init_Actvtn_St : Constant  Value=0
  TrlrAidMde_D_Rq : Constant  Value=0
  bus_creator : BusCreator  Inputs=15
  out_port : Outport
  wires:
  bus_creator/1 -> out_port/1  "Subsystem2"
  OnbChrgClearAll_B_Rq/1 -> bus_creator/1  "OnbChrgClearAll_B_Rq"
  OnbChrgGoTDelete_B_Rq/1 -> bus_creator/2  "OnbChrgGoTDelete_B_Rq"
  OnbChrgGoTElement_D_Rq/1 -> bus_creator/3  "OnbChrgGoTElement_D_Rq"
  OnbChrgGoTExtHtr_D_Rq/1 -> bus_creator/4  "OnbChrgGoTExtHtr_D_Rq"
  OnbChrgGoTHr_T_Rq/1 -> bus_creator/5  "OnbChrgGoTHr_T_Rq"
  OnbChrgGoTMnte_D_Rq/1 -> bus_creator/6  "OnbChrgGoTMnte_D_Rq"
  OnbChrgGoTOn_D_Rq/1 -> bus_creator/7  "OnbChrgGoTOn_D_Rq"
  OnbChrgGoTPrcond_D_Rq/1 -> bus_creator/8  "OnbChrgGoTPrcond_D_Rq"
  OnbChrgGoTTouch_D_Rq/1 -> bus_creator/9  "OnbChrgGoTTouch_D_Rq"
  OnbChrgGoTUpdate_B_Rq/1 -> bus_creator/10  "OnbChrgGoTUpdate_B_Rq"
  OtaTrg_D_Stat/1 -> bus_creator/11  "OtaTrg_D_Stat"
  PaakMyKey_D_Rq/1 -> bus_creator/12  "PaakMyKey_D_Rq"
  TCU_Final_Actvtn_St/1 -> bus_creator/13  "TCU_Final_Actvtn_St"
  TCU_Init_Actvtn_St/1 -> bus_creator/14  "TCU_Init_Actvtn_St"
  TrlrAidMde_D_Rq/1 -> bus_creator/15  "TrlrAidMde_D_Rq"

== system P702_NI_SoftECU/Output/Subsystem2/CAN_Signal/GWM/Other_GWMTx/ActiveFrontStrg_Stat2_FD1 ==
  SteWhlRelCalib_An_Sns : Constant  Value=0
  SteWhlRelCalib_T_Actl : Constant  Value=0
  bus_creator : BusCreator  Inputs=2
  out_port : Outport
  wires:
  bus_creator/1 -> out_port/1  "Subsystem2"
  SteWhlRelCalib_An_Sns/1 -> bus_creator/1  "SteWhlRelCalib_An_Sns"
  SteWhlRelCalib_T_Actl/1 -> bus_creator/2  "SteWhlRelCalib_T_Actl"

== system P702_NI_SoftECU/Output/Subsystem2/CAN_Signal/GWM/Other_GWMTx/ActiveFrontStrg_Stat_FD1 ==
  SteWhlBrkAnActl_No_Cnt : Constant  Value=0
  SteWhlBrkAnActl_No_Cs : Constant  Value=0
  SteWhlBrkOffst_An_Actl : Constant  Value=0
  SteWhlOffstRq_D_Stat : Constant  Value=0
  SteWhlOffst_An_TotActl : Constant  Value=0
  bus_creator : BusCreator  Inputs=5
  out_port : Outport
  wires:
  bus_creator/1 -> out_port/1  "Subsystem2"
  SteWhlBrkAnActl_No_Cnt/1 -> bus_creator/1  "SteWhlBrkAnActl_No_Cnt"
  SteWhlBrkAnActl_No_Cs/1 -> bus_creator/2  "SteWhlBrkAnActl_No_Cs"
  SteWhlBrkOffst_An_Actl/1 -> bus_creator/3  "SteWhlBrkOffst_An_Actl"
  SteWhlOffstRq_D_Stat/1 -> bus_creator/4  "SteWhlOffstRq_D_Stat"
  SteWhlOffst_An_TotActl/1 -> bus_creator/5  "SteWhlOffst_An_TotActl"

== system P702_NI_SoftECU/Output/Subsystem2/CAN_Signal/GWM/Other_GWMTx/AllTerrainControlData_FD1 ==
  SelDrvMdeCnt_D_Stat : Constant  Value=0
  SelDrvMdeSwtchOk_D_Stat : Constant  Value=0
  SelDrvMdeSwtch_D_Stat : Constant  Value=0
  SelDrvMdeSwtch_No_Actl : Constant  Value=0
  bus_creator : BusCreator  Inputs=4
  out_port : Outport
  wires:
  bus_creator/1 -> out_port/1  "Subsystem2"
  SelDrvMdeCnt_D_Stat/1 -> bus_creator/1  "SelDrvMdeCnt_D_Stat"
  SelDrvMdeSwtchOk_D_Stat/1 -> bus_creator/2  "SelDrvMdeSwtchOk_D_Stat"
  SelDrvMdeSwtch_D_Stat/1 -> bus_creator/3  "SelDrvMdeSwtch_D_Stat"
  SelDrvMdeSwtch_No_Actl/1 -> bus_creator/4  "SelDrvMdeSwtch_No_Actl"

== system P702_NI_SoftECU/Output/Subsystem2/CAN_Signal/GWM/Other_GWMTx/All_Terrain_Data_FD1 ==
  TerrMde_D_RqDrv : Constant  Value=0
  TerrStat_D_RqDsply : Constant  Value=0
  bus_creator : BusCreator  Inputs=2
  out_port : Outport
  wires:
  bus_creator/1 -> out_port/1  "Subsystem2"
  TerrMde_D_RqDrv/1 -> bus_creator/1  "TerrMde_D_RqDrv"
  TerrStat_D_RqDsply/1 -> bus_creator/2  "TerrStat_D_RqDsply"

== system P702_NI_SoftECU/Output/Subsystem2/CAN_Signal/GWM/Other_GWMTx/BCM_Lamp_Stat_FD1 ==
  BrkWarnInd_B_Rq : Constant  Value=0
  Brk_Fluid_Lvl_Low : Constant  Value=0
  Courtesy_BSave_Stat : Constant  Value=0
  Courtesy_Delay_Status : Constant  Value=0
  CrnrLghtLeft_Pc_Rq : Constant  Value=0
  CrnrLghtRight_Pc_Rq : Constant  Value=0
  DayRnngLampOn_B_Stat : Constant  Value=0
  DrTgateLck_D_Stat : Constant  Value=0
  Dr_Courtesy_Light_Stat : Constant  Value=0
  HeadLampLoActv_B_Stat : Constant  Value=0
  HeadLampLoFlOn_B_Stat : Constant  Value=0
  HeadLampLoFrOn_B_Stat : Constant  Value=0
  HeadLampLoOut_B_Stat : Constant  Value=0
  HeadLghtHiFdbck_D_Stat : Constant  Value=0
  HeadLghtHiOn_B_Stat : Constant  Value=0
  HeadLghtSwtch_D_Stat : Constant  Value=0
  Headlamp_On_Wrning_Cmd : Constant  Value=0
  HomeSafeLtChime_B_Rq : Constant  Value=0
  Illuminated_Entry_Stat : Constant  Value=0
  ImpactEvntFdbck_D_Stat : Constant  Value=0
  KeyInIgnWarn_B_Cmd : Constant  Value=0
  Park_Brake_Chime_Rqst : Constant  Value=0
  PerimeterAlarmChimeRq : Constant  Value=0
  Perimeter_Alarm_Status : Constant  Value=0
  PrkLght_D_Stat : Constant  Value=0
  PrkLightChime_B_Rq : Constant  Value=0
  PudLampDrv_D_Rq : Constant  Value=0
  PudLampPsngr_D_Rq : Constant  Value=0
  PudLamp_D_Rq : Constant  Value=0
  ReducedGuard_D_Stat : Constant  Value=0
  RvrseLghtOn_B_Stat : Constant  Value=0
  StopLghtOn_B_Stat : Constant  Value=0
  TrnNotInPrkChime_B_Rq : Constant  Value=0
  WndwGlbl_D_Cmd : Constant  Value=0
  WrlssAcsyChrgInhbt_B_Rq : Constant  Value=0
  bus_creator : BusCreator  Inputs=35
  out_port : Outport
  wires:
  bus_creator/1 -> out_port/1  "Subsystem2"
  BrkWarnInd_B_Rq/1 -> bus_creator/1  "BrkWarnInd_B_Rq"
  Brk_Fluid_Lvl_Low/1 -> bus_creator/2  "Brk_Fluid_Lvl_Low"
  Courtesy_BSave_Stat/1 -> bus_creator/3  "Courtesy_BSave_Stat"
  Courtesy_Delay_Status/1 -> bus_creator/4  "Courtesy_Delay_Status"
  CrnrLghtLeft_Pc_Rq/1 -> bus_creator/5  "CrnrLghtLeft_Pc_Rq"
  CrnrLghtRight_Pc_Rq/1 -> bus_creator/6  "CrnrLghtRight_Pc_Rq"
  DayRnngLampOn_B_Stat/1 -> bus_creator/7  "DayRnngLampOn_B_Stat"
  DrTgateLck_D_Stat/1 -> bus_creator/8  "DrTgateLck_D_Stat"
  Dr_Courtesy_Light_Stat/1 -> bus_creator/9  "Dr_Courtesy_Light_Stat"
  HeadLampLoActv_B_Stat/1 -> bus_creator/10  "HeadLampLoActv_B_Stat"
  HeadLampLoFlOn_B_Stat/1 -> bus_creator/11  "HeadLampLoFlOn_B_Stat"
  HeadLampLoFrOn_B_Stat/1 -> bus_creator/12  "HeadLampLoFrOn_B_Stat"
  HeadLampLoOut_B_Stat/1 -> bus_creator/13  "HeadLampLoOut_B_Stat"
  HeadLghtHiFdbck_D_Stat/1 -> bus_creator/14  "HeadLghtHiFdbck_D_Stat"
  HeadLghtHiOn_B_Stat/1 -> bus_creator/15  "HeadLghtHiOn_B_Stat"
  HeadLghtSwtch_D_Stat/1 -> bus_creator/16  "HeadLghtSwtch_D_Stat"
  Headlamp_On_Wrning_Cmd/1 -> bus_creator/17  "Headlamp_On_Wrning_Cmd"
  HomeSafeLtChime_B_Rq/1 -> bus_creator/18  "HomeSafeLtChime_B_Rq"
  Illuminated_Entry_Stat/1 -> bus_creator/19  "Illuminated_Entry_Stat"
  ImpactEvntFdbck_D_Stat/1 -> bus_creator/20  "ImpactEvntFdbck_D_Stat"
  KeyInIgnWarn_B_Cmd/1 -> bus_creator/21  "KeyInIgnWarn_B_Cmd"
  Park_Brake_Chime_Rqst/1 -> bus_creator/22  "Park_Brake_Chime_Rqst"
  PerimeterAlarmChimeRq/1 -> bus_creator/23  "PerimeterAlarmChimeRq"
  Perimeter_Alarm_Status/1 -> bus_creator/24  "Perimeter_Alarm_Status"
  PrkLght_D_Stat/1 -> bus_creator/25  "PrkLght_D_Stat"
  PrkLightChime_B_Rq/1 -> bus_creator/26  "PrkLightChime_B_Rq"
  PudLampDrv_D_Rq/1 -> bus_creator/27  "PudLampDrv_D_Rq"
  PudLampPsngr_D_Rq/1 -> bus_creator/28  "PudLampPsngr_D_Rq"
  PudLamp_D_Rq/1 -> bus_creator/29  "PudLamp_D_Rq"
  ReducedGuard_D_Stat/1 -> bus_creator/30  "ReducedGuard_D_Stat"
  RvrseLghtOn_B_Stat/1 -> bus_creator/31  "RvrseLghtOn_B_Stat"
  StopLghtOn_B_Stat/1 -> bus_creator/32  "StopLghtOn_B_Stat"
  TrnNotInPrkChime_B_Rq/1 -> bus_creator/33  "TrnNotInPrkChime_B_Rq"
  WndwGlbl_D_Cmd/1 -> bus_creator/34  "WndwGlbl_D_Cmd"
  WrlssAcsyChrgInhbt_B_Rq/1 -> bus_creator/35  "WrlssAcsyChrgInhbt_B_Rq"

== system P702_NI_SoftECU/Output/Subsystem2/CAN_Signal/GWM/Other_GWMTx/BatteryCharge_Data2_FD1 ==
  ChrgCrdLck_D_Falt : Constant  Value=0
  bus_creator : BusCreator  Inputs=1
  out_port : Outport
  wires:
  bus_creator/1 -> out_port/1  "Subsystem2"
  ChrgCrdLck_D_Falt/1 -> bus_creator/1  "ChrgCrdLck_D_Falt"
